simulink model "optimal_observer_model"  (R2023b)
settings: Solver=VariableStepAuto  StartTime=0.0  StopTime=15  RelTol=1e-3
values from neighbouring files (symbols this model uses):
  Kr = -inv((sys_c.C-sys_c.D*K)*inv(sys_d.A-eye(2)-sys_d.B*K)*sys_d.B-sys_c.D)    [optimal_observer_script.m]
  L = place(sys_d.A', sys_d.C', P_o)'    [optimal_observer_script.m]
  sys_c = ss(A, B, C, D)    [optimal_observer_script.m]    (also in state_space_derivation.m)
  sys_d = c2d(sys_c, Ts)    [optimal_observer_script.m]    (also in state_space_derivation.m)
undefined symbols (not defined in the file or in its folder): K
settings Model: Creator=charl  LastModifiedBy=charl

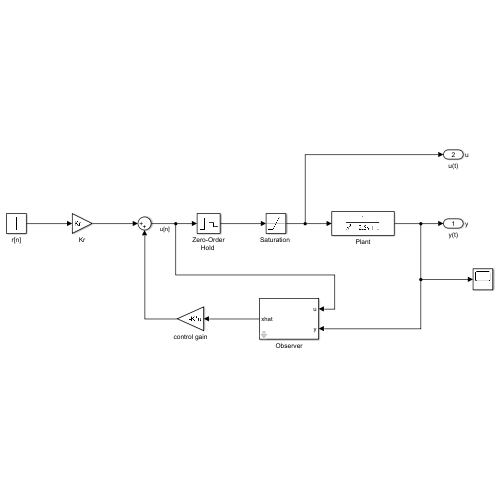
[thumbnail: Simulink's stored preview of the top-level diagram]
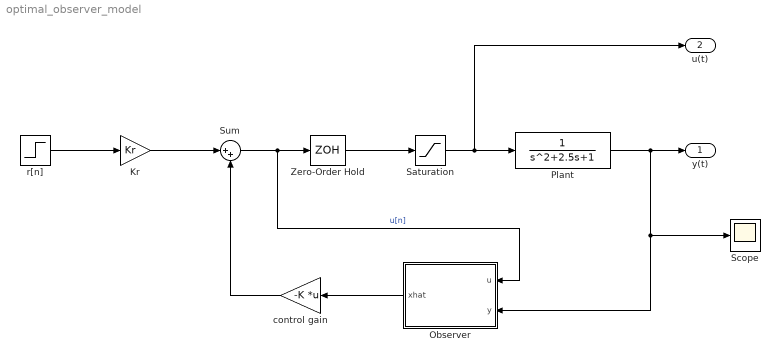
== system optimal_observer_model ==
  " Observer " : Subsystem
  Kr : Gain  Gain=Kr
  Plant : TransferFcn  Denominator=[1 2.5 1]
  "Saturation " : Saturate  UpperLimit=5  LowerLimit=0
  Scope : Scope
  Sum : Sum  Inputs=|++
  "Zero-Order Hold " : ZeroOrderHold  SampleTime=-1
  control gain : Gain  Gain=-K  Multiplication=Matrix(K*u)
  r[n] : Step  Time=0  After=2.5  SampleTime=0
  y(t) : Outport  SignalName=y
  u(t) : Outport  Port=2  SignalName=u
  wires:
  r[n]/1 -> Kr/1
  Kr/1 -> Sum/1
  Sum/1 -> " Observer "/1(u), "Zero-Order Hold "/1  "u[n]"
  "Zero-Order Hold "/1 -> "Saturation "/1
  control gain/1 -> Sum/2
  "Saturation "/1 -> u(t)/1, Plant/1
  Plant/1 -> Scope/1, " Observer "/2(y), y(t)/1
  " Observer "/1(xhat) -> control gain/1

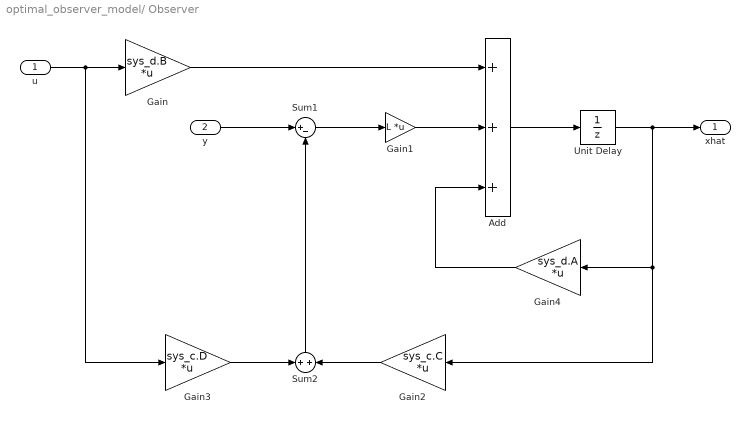
== system optimal_observer_model/ Observer  ==
  u : Inport
  y : Inport  Port=2
  Add : Sum  Inputs=+++
  Gain : Gain  Gain=sys_d.B  Multiplication=Matrix(K*u)
  Gain1 : Gain  Gain=L  Multiplication=Matrix(K*u) (u vector)
  Gain2 : Gain  Gain=sys_c.C  Multiplication=Matrix(K*u)
  Gain3 : Gain  Gain=sys_c.D  Multiplication=Matrix(K*u)
  Gain4 : Gain  Gain=sys_d.A  Multiplication=Matrix(K*u)
  Sum1 : Sum  Inputs=|+-
  Sum2 : Sum  Inputs=+|+
  "Unit Delay " : UnitDelay  SampleTime=-1  HasFrameUpgradeWarning=on
  xhat : Outport
  wires:
  Sum2/1 -> Sum1/2
  Sum1/1 -> Gain1/1
  "Unit Delay "/1 -> xhat/1, Gain4/1, Gain2/1
  u/1 -> Gain3/1, Gain/1
  Gain/1 -> Add/1
  Gain1/1 -> Add/2
  Add/1 -> "Unit Delay "/1
  y/1 -> Sum1/1
  Gain2/1 -> Sum2/2
  Gain4/1 -> Add/3
  Gain3/1 -> Sum2/1
